simulink model "lab06q1"  (Simulink 7.1)
settings: Solver=ode45  StartTime=0.0  StopTime=100  RelTol=1e-3
InitFcn:
  | RC = 2;
  | K= (1/2);
  | 
  | 
  | A = [(-1/RC)*(2-K) (1/RC)*K (-1/RC);(1/RC)*K (1/RC)*K (-1/RC);(1/(2*RC))*(1+2*K) (1/(2*RC))*(1+2*K) (-1/RC)]
  | 
  | B = [(1/RC)*(2-K);(-1/RC)*K;(-1/RC)*K]
  | 
  | C = [-(1+K) -(1+K) 0;1 0 0;0 1 0;0 0 1]
  | 
  | D = [(1+K);0;0;0]
libraries: simulink x9
settings Model: Creator=ALUNO  LastModifiedBy=ALUNO

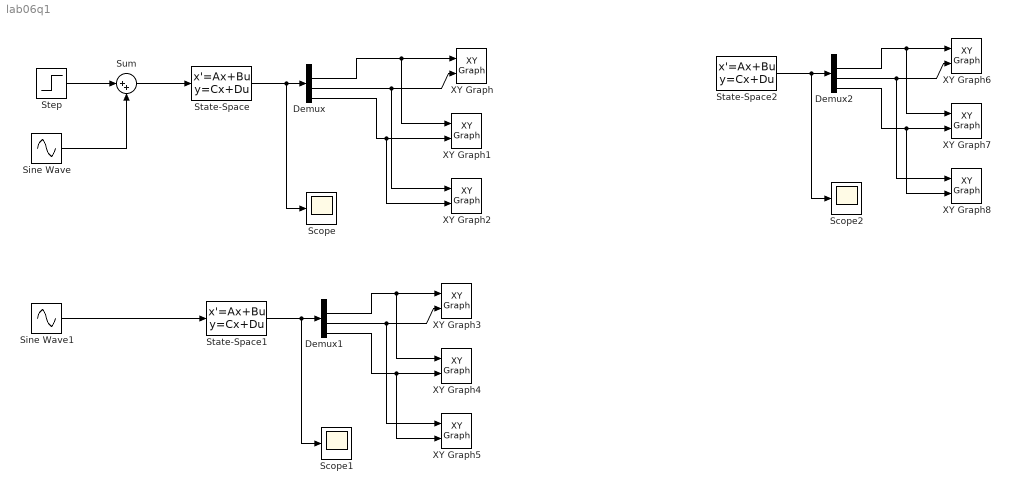
== system lab06q1 ==
  Demux : Demux
  Demux1 : Demux
  Demux2 : Demux
  Scope : Scope
  Scope1 : Scope
  Scope2 : Scope
      settings: SaveName=ScopeData2
  Sine Wave : Sin  Frequency=4  SampleTime=0
  Sine Wave1 : Sin  Frequency=0.5  SampleTime=0
  State-Space : StateSpace  A=A  B=B  C=C  D=D
  State-Space1 : StateSpace  A=A  B=B  C=C  D=D
  State-Space2 : StateSpace  A=A  B=B  C=C  D=D  X0=[4;-3;8]
  Step : Step  Time=0  SampleTime=0
  Sum : Sum  Inputs=|++  OutDataType=sfix(16)  OutScaling=2^0
  XY Graph{,1..5} (6 alike) : simulink/Sinks/XY Graph  SystemSampleTime=-1  xmin=-2  xmax=2  ymin=-2  ymax=2  st=-1
  XY Graph6 : simulink/Sinks/XY Graph  SystemSampleTime=-1  xmin=-5  xmax=5  ymin=-5  ymax=5  st=-1
  XY Graph7 : simulink/Sinks/XY Graph  SystemSampleTime=-1  xmin=-5  xmax=5  ymin=-5  ymax=5  st=-1
  XY Graph8 : simulink/Sinks/XY Graph  SystemSampleTime=-1  xmin=-5  xmax=5  ymin=-5  ymax=5  st=-1
  wires:
  Step/1 -> Sum/1
  Sum/1 -> State-Space/1
  State-Space/1 -> Demux/1, Scope/1
  Demux/2 -> XY Graph/1, XY Graph1/1
  Demux/3 -> XY Graph/2, XY Graph2/1
  State-Space1/1 -> Demux1/1, Scope1/1
  Demux1/2 -> XY Graph3/1, XY Graph4/1
  Demux1/3 -> XY Graph3/2, XY Graph5/1
  Demux1/4 -> XY Graph4/2, XY Graph5/2
  Sine Wave1/1 -> State-Space1/1
  Demux/4 -> XY Graph1/2, XY Graph2/2
  Sine Wave/1 -> Sum/2
  State-Space2/1 -> Demux2/1, Scope2/1
  Demux2/2 -> XY Graph6/1, XY Graph7/1
  Demux2/3 -> XY Graph6/2, XY Graph8/1
  Demux2/4 -> XY Graph7/2, XY Graph8/2
